simulink model "export_data"  (R2022b)
settings: Solver=VariableStepAuto  StartTime=0.0  StopTime=10.0  RelTol=1e-3
settings Model: Creator=craft  LastModifiedBy=craft

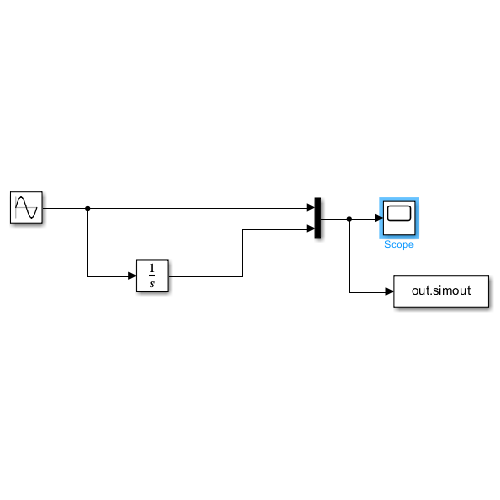
[thumbnail: Simulink's stored preview of the top-level diagram]
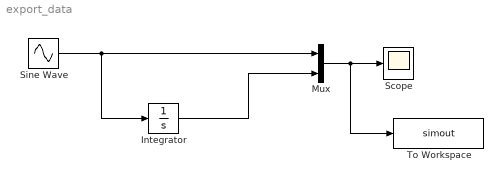
== system export_data ==
  Integrator : Integrator
  Mux : Mux  Inputs=2
  Scope : Scope
  Sine Wave : Sin  SampleTime=0
  To Workspace : ToWorkspace  VariableName=simout  SaveFormat=Structure With Time  SampleTime=-1
  wires:
  Sine Wave/1 -> Integrator/1, Mux/1
  Mux/1 -> To Workspace/1, Scope/1
  Integrator/1 -> Mux/2
